simulink model "subsystem2"  (Simulink 7.5)
settings: Solver=ode45  StartTime=0.0  StopTime=10.0  RelTol=1e-3
settings Model: Creator=lm  LastModifiedBy=lm

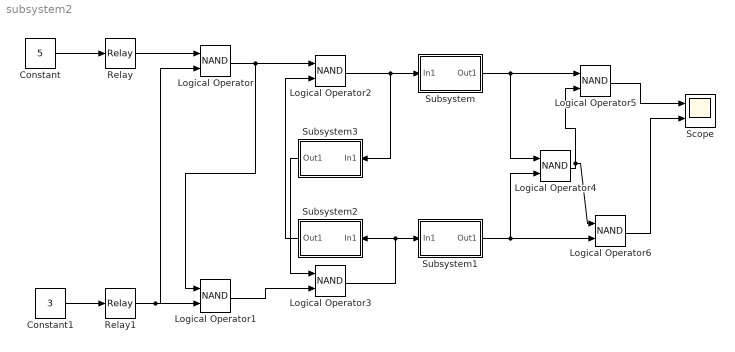
== system subsystem2 ==
  Constant : Constant  Value=5  OutDataType=fixdt(1, 16)  OutScaling=2^0
  Constant1 : Constant  Value=3  OutDataType=fixdt(1, 16)  OutScaling=2^0
  Logical Operator : Logic  Operator=NAND  AllPortsSameDT=off  LogicDataType=fixdt(0, 8)
  Logical Operator{1..6} (6 alike) : Logic  Operator=NAND  AllPortsSameDT=off  OutDataTypeMode=boolean  LogicDataType=fixdt(0, 8)  OutDataTypeStr=boolean
  Relay : Relay  OnSwitchValue=0.001  OffSwitchValue=-0.001  OutDataType=fixdt(1, 16)  OutScaling=2^0
  Relay1 : Relay  OnSwitchValue=0.5  OffSwitchValue=0.01  OnOutputValue=0  OffOutputValue=1  OutDataType=fixdt(1, 16)  OutScaling=2^0
  Scope : Scope  NumInputPorts=2
      settings: YMin=-5~-5  YMax=5~5
  Subsystem : Subsystem
  Subsystem1 : Subsystem
  Subsystem2 : Subsystem
  Subsystem3 : Subsystem
  wires:
  Relay/1 -> Logical Operator/1
  Relay1/1 -> Logical Operator1/2, Logical Operator/2
  Logical Operator/1 -> Logical Operator1/1, Logical Operator2/1
  Subsystem2/1(Out1) -> Logical Operator2/2
  Subsystem3/1(Out1) -> Logical Operator3/1
  Logical Operator1/1 -> Logical Operator3/2
  Logical Operator3/1 -> Subsystem1/1(In1), Subsystem2/1(In1)
  Logical Operator2/1 -> Subsystem/1(In1), Subsystem3/1(In1)
  Subsystem/1(Out1) -> Logical Operator5/1, Logical Operator4/1
  Subsystem1/1(Out1) -> Logical Operator6/2, Logical Operator4/2
  Logical Operator4/1 -> Logical Operator6/1, Logical Operator5/2
  Logical Operator5/1 -> Scope/1
  Logical Operator6/1 -> Scope/2
  Constant/1 -> Relay/1
  Constant1/1 -> Relay1/1

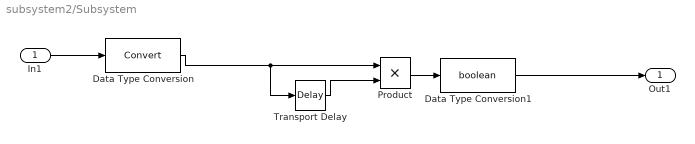
== system subsystem2/Subsystem ==
  In1 : Inport  OutDataType=fixdt(1, 16)  OutScaling=2^0
  Data Type Conversion : DataTypeConversion  OutDataType=fixdt(1, 16)  OutScaling=2^0
  Data Type Conversion1 : DataTypeConversion  OutDataTypeMode=boolean  OutDataType=fixdt(1, 16)  OutScaling=2^0  OutDataTypeStr=boolean
  Product : Product  OutDataType=fixdt(1, 16)  OutScaling=2^0  RndMeth=Zero
  Transport Delay : TransportDelay  DelayTime=7e-3
  Out1 : Outport  OutDataType=fixdt(1, 16)  OutScaling=2^0
  wires:
  Transport Delay/1 -> Product/2
  Data Type Conversion/1 -> Transport Delay/1, Product/1
  In1/1 -> Data Type Conversion/1
  Product/1 -> Data Type Conversion1/1
  Data Type Conversion1/1 -> Out1/1

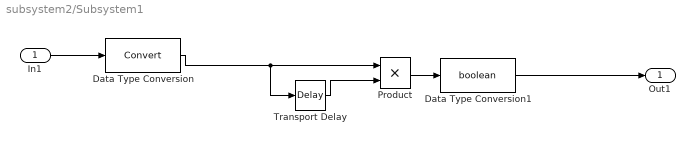
== system subsystem2/Subsystem1 ==
  In1 : Inport  OutDataType=fixdt(1, 16)  OutScaling=2^0
  Data Type Conversion : DataTypeConversion  OutDataType=fixdt(1, 16)  OutScaling=2^0
  Data Type Conversion1 : DataTypeConversion  OutDataTypeMode=boolean  OutDataType=fixdt(1, 16)  OutScaling=2^0  OutDataTypeStr=boolean
  Product : Product  OutDataType=fixdt(1, 16)  OutScaling=2^0  RndMeth=Zero
  Transport Delay : TransportDelay  DelayTime=7e-3
  Out1 : Outport  OutDataType=fixdt(1, 16)  OutScaling=2^0
  wires:
  Data Type Conversion1/1 -> Out1/1
  Product/1 -> Data Type Conversion1/1
  In1/1 -> Data Type Conversion/1
  Data Type Conversion/1 -> Product/1, Transport Delay/1
  Transport Delay/1 -> Product/2

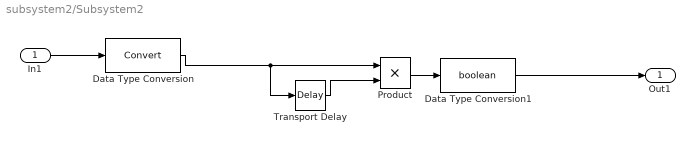
== system subsystem2/Subsystem2 ==
  In1 : Inport  OutDataType=fixdt(1, 16)  OutScaling=2^0
  Data Type Conversion : DataTypeConversion  OutDataType=fixdt(1, 16)  OutScaling=2^0
  Data Type Conversion1 : DataTypeConversion  OutDataTypeMode=boolean  OutDataType=fixdt(1, 16)  OutScaling=2^0  OutDataTypeStr=boolean
  Product : Product  OutDataType=fixdt(1, 16)  OutScaling=2^0  RndMeth=Zero
  Transport Delay : TransportDelay  DelayTime=3e-3
  Out1 : Outport  OutDataType=fixdt(1, 16)  OutScaling=2^0
  wires:
  Transport Delay/1 -> Product/2
  Data Type Conversion/1 -> Transport Delay/1, Product/1
  In1/1 -> Data Type Conversion/1
  Product/1 -> Data Type Conversion1/1
  Data Type Conversion1/1 -> Out1/1

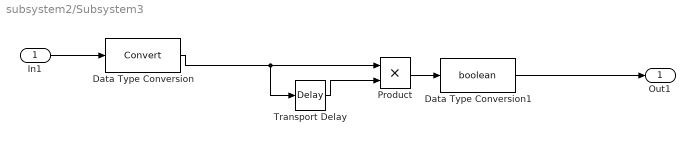
== system subsystem2/Subsystem3 ==
  In1 : Inport  OutDataType=fixdt(1, 16)  OutScaling=2^0
  Data Type Conversion : DataTypeConversion  OutDataType=fixdt(1, 16)  OutScaling=2^0
  Data Type Conversion1 : DataTypeConversion  OutDataTypeMode=boolean  OutDataType=fixdt(1, 16)  OutScaling=2^0  OutDataTypeStr=boolean
  Product : Product  OutDataType=fixdt(1, 16)  OutScaling=2^0  RndMeth=Zero
  Transport Delay : TransportDelay  DelayTime=3e-3
  Out1 : Outport  OutDataType=fixdt(1, 16)  OutScaling=2^0
  wires:
  Data Type Conversion1/1 -> Out1/1
  Product/1 -> Data Type Conversion1/1
  In1/1 -> Data Type Conversion/1
  Data Type Conversion/1 -> Product/1, Transport Delay/1
  Transport Delay/1 -> Product/2
